simulink model "UberCase_cs"  (R2015b)
settings: Solver=ode5  SolverMode=SingleTasking  StartTime=0.0  StopTime=inf  FixedStep=1/100  RelTol=1e-3
PreLoadFcn:
  | mbxruntime.callbacks.PreLoadFcn(bdroot);
PostLoadFcn:
  | mbxruntime.callbacks.PostLoadFcn(bdroot);
InitFcn:
  | mbxruntime.callbacks.InitFcn(bdroot);
StartFcn:
  | mbxruntime.callbacks.StartFcn(bdroot);
StopFcn:
  | mbxruntime.callbacks.StopFcn(bdroot);
model workspace (MAT data in the model file):
  mbox_table : struct (value not decoded)
  model_closed = 0
  sim_status = 0
undefined symbols (not defined in the file or in its folder): DiscIntNeverNeededParam, InitImageOutputDir, mbxruntime, tabledata
libraries: PreScanSimulinkLibrary x32, simulink_extras x2, PreScanUsefulBlocks x1
(part 3 of 6)

== system UberCase_cs/STATE_Mazda_RX8_2_bus/ENABLED ==
  STATE_Mazda_RX8_2_bus : Inport  Tag=inport/StatePort  OutDataTypeStr=Bus: PRESCAN_STATEACTUATORDATA  PortDimensions=1  SampleTime=1/100  BusOutputAsStruct=on
  Actuator : S-Function  FunctionName=sfun_StateActuator  Parameters=UniqueID, TimeStep  SFunctionDeploymentMode=off  EnableBusSupport=off  mask(PreScan Sink Block: State){UniqueID=564, TimeStep=1/100}
      mask prompts: UniqueID "Auto-Assigned: Unique ID"; TimeStep "Auto-Assigned: Upload Period [s]"
      mask help:
      | The Actor State contains a vector signal of size (9x1), containing the following signals:
      |
      | -  Position    	(x,y,z)             	[m]
      | -  Velocity    	(vx,vy,vz)         	[m/s]
      | -  Angles       	(Roll, Pitch, Yaw)	[rad]
      |
      | The Actor state is defined in the global axis system.
      | The state is superponed on the Initial position defined in the GUI.
      |
      | For more information, please click Help.
      mask Help: eval('openHelp(222)')
      mask Display: image(imread('State.png'))
  wires:
  STATE_Mazda_RX8_2_bus/1 -> Actuator/1

== system UberCase_cs/STATE_Toyota_Previa_1_bus/DISABLED ==
  STATE_Toyota_Previa_1_bus : Inport  Tag=inport/StatePort  OutDataTypeStr=Bus: PRESCAN_STATEACTUATORDATA  PortDimensions=1  SampleTime=1/100  BusOutputAsStruct=on
  TRM1 : Terminator
  wires:
  STATE_Toyota_Previa_1_bus/1 -> TRM1/1

== system UberCase_cs/STATE_Toyota_Previa_1_bus/ENABLED ==
  STATE_Toyota_Previa_1_bus : Inport  Tag=inport/StatePort  OutDataTypeStr=Bus: PRESCAN_STATEACTUATORDATA  PortDimensions=1  SampleTime=1/100  BusOutputAsStruct=on
  Actuator : S-Function  FunctionName=sfun_StateActuator  Parameters=UniqueID, TimeStep  SFunctionDeploymentMode=off  EnableBusSupport=off  mask(PreScan Sink Block: State){UniqueID=665, TimeStep=1/100}
      mask prompts: UniqueID "Auto-Assigned: Unique ID"; TimeStep "Auto-Assigned: Upload Period [s]"
      mask help:
      | The Actor State contains a vector signal of size (9x1), containing the following signals:
      |
      | -  Position    	(x,y,z)             	[m]
      | -  Velocity    	(vx,vy,vz)         	[m/s]
      | -  Angles       	(Roll, Pitch, Yaw)	[rad]
      |
      | The Actor state is defined in the global axis system.
      | The state is superponed on the Initial position defined in the GUI.
      |
      | For more information, please click Help.
      mask Help: eval('openHelp(222)')
      mask Display: image(imread('State.png'))
  wires:
  STATE_Toyota_Previa_1_bus/1 -> Actuator/1

== system UberCase_cs/STATE_Uber_Car_bus/DISABLED ==
  STATE_Uber_Car_bus : Inport  Tag=inport/StatePort  OutDataTypeStr=Bus: PRESCAN_STATEACTUATORDATA  PortDimensions=1  SampleTime=1/100  BusOutputAsStruct=on
  TRM1 : Terminator
  wires:
  STATE_Uber_Car_bus/1 -> TRM1/1

== system UberCase_cs/STATE_Uber_Car_bus/ENABLED ==
  STATE_Uber_Car_bus : Inport  Tag=inport/StatePort  OutDataTypeStr=Bus: PRESCAN_STATEACTUATORDATA  PortDimensions=1  SampleTime=1/100  BusOutputAsStruct=on
  Actuator : S-Function  FunctionName=sfun_StateActuator  Parameters=UniqueID, TimeStep  SFunctionDeploymentMode=off  EnableBusSupport=off  mask(PreScan Sink Block: State){UniqueID=372, TimeStep=1/100}
      mask prompts: UniqueID "Auto-Assigned: Unique ID"; TimeStep "Auto-Assigned: Upload Period [s]"
      mask help:
      | The Actor State contains a vector signal of size (9x1), containing the following signals:
      |
      | -  Position    	(x,y,z)             	[m]
      | -  Velocity    	(vx,vy,vz)         	[m/s]
      | -  Angles       	(Roll, Pitch, Yaw)	[rad]
      |
      | The Actor state is defined in the global axis system.
      | The state is superponed on the Initial position defined in the GUI.
      |
      | For more information, please click Help.
      mask Help: eval('openHelp(222)')
      mask Display: image(imread('State.png'))
  wires:
  STATE_Uber_Car_bus/1 -> Actuator/1

== system UberCase_cs/Toyota_Previa_1/DISABLED ==
  SELF_Toyota_Previa_1 : Inport  Tag=inport/SelfPort  OutDataTypeStr=Bus: PRESCAN_SELFSENSORDATA  PortDimensions=1  SampleTime=1/100  BusOutputAsStruct=on
  GND1 : Subsystem
  TRM1 : Terminator
  STATE_Toyota_Previa_1_bus : Outport  Tag=outport/StatePort  OutDataTypeStr=Bus: PRESCAN_STATEACTUATORDATA  PortDimensions=1  SampleTime=1/100
  wires:
  SELF_Toyota_Previa_1/1 -> TRM1/1
  GND1/1(bus) -> STATE_Toyota_Previa_1_bus/1

== system UberCase_cs/Toyota_Previa_1/ENABLED ==
  SELF_Toyota_Previa_1 : Inport  Tag=inport/SelfPort  OutDataTypeStr=Bus: PRESCAN_SELFSENSORDATA  PortDimensions=1  SampleTime=1/100  BusOutputAsStruct=on
  Dynamics_Empty : Subsystem  Tag=Dynamics_Empty
      mask Help: eval('openHelp(202)')
      mask Display: port_label('output', 1, 'State');text(0,0,' Empty\n')
  SELF_Demux : Subsystem  Tag=demux/SelfPort  mask(PreScan Demux Block:){}
      mask help:
      | The SELF port shows (state) information of the actor itself. The outputs are position in the experiment's axis system and the GPS coordinates, and the object's absolute velocity and compass heading.
      |
      | For more information, please click Help.
      settings: DeleteFcn=PreScanBlockDeleteFcn;
      mask Help: eval('openHelp(462)')
      mask Display:
      | port_label('output',1,'x [m]')
      | port_label('output',2,'y [m]')
      | port_label('output',3,'z [m]','texmode','on')
      | port_label('output',4,'Rotx [deg]','texmode','on')
      | port_label('output',5,'Roty [deg]','texmode','on')
      | port_label('output',6,'Rotz [deg]','texmode','on')
      | port_label('output',7,'GPS lat [deg]','texmode','on')
      | port_label('output',8,'GPS long [deg]','texmode','on')
      | port_label('output',9,'GPS alt [m]','texmode','on')
      | port_label('output',10,'Velocity [m/s]')
      | port_label('output',11,'Heading [deg]')
      | port_label('output',12,'Yaw rate [deg/s]')
  STATE_Toyota_Previa_1 : Subsystem  Tag=mux/StatePort  Priority=0  LoadFcn=load PrescanStateActuatorData  mask(PreScan Sink Block: State){x0=82.046318054199219, y0=122.2374267578125, z0=0.71, Roll0=0, Pitch0=0, Yaw0=90, TimeStep=1/100}
      mask prompts: x0 "Ini x-position VEHICLE wrt GLOBAL axis system [m]"; y0 "Ini y-position VEHICLE wrt GLOBAL axis system [m]"; z0 "Ini z-position VEHICLE wrt GLOBAL axis system [m]"; Roll0 "Ini roll-angle BODY wrt VEHICLE axis system [deg]"; Pitch0 "Ini pitch-angle BODY wrt VEHICLE axis system [deg]"; Yaw0 "Ini yaw-angle VEHICLE wrt GLOBAL axis system [deg]"; TimeStep "Auto-Assigned: Upload Period [s]"
      mask help:
      | The Actor State contains a vector signal of size (9x1), containing the following signals:
      |
      | -  Position                  (x,y,z)                                     [m]
      | -  Velocity                  (vx,vy,vz)                               [m/s]
      | -  Angles                    (Roll, Pitch, Yaw)                   [rad]
      |
      | The Actor state is defined in the global axis system.
      | The state is superponed on the Initial position defined in the GUI.
      |
      | For more information, please click Help.
      settings: DeleteFcn=PreScanBlockDeleteFcn;
      mask Help: eval('openHelp(222)')
      mask Display: image(imread('State.png'))
  Terminator_{1..12} (12 alike) : Terminator
  STATE_Toyota_Previa_1_bus : Outport  Tag=outport/StatePort  OutDataTypeStr=Bus: PRESCAN_STATEACTUATORDATA  PortDimensions=1  SampleTime=1/100
  wires:
  STATE_Toyota_Previa_1/1(StateBus) -> STATE_Toyota_Previa_1_bus/1
  SELF_Toyota_Previa_1/1 -> SELF_Demux/1(SELF)
  Dynamics_Empty/1(State) -> STATE_Toyota_Previa_1/1(State)
  SELF_Demux/1(x [m]) -> Terminator_1/1
  SELF_Demux/2(y [m]) -> Terminator_2/1
  SELF_Demux/3(z [m]) -> Terminator_3/1
  SELF_Demux/4(rotx [deg]) -> Terminator_4/1
  SELF_Demux/5(roty [deg]) -> Terminator_5/1
  SELF_Demux/6(rotz [deg]) -> Terminator_6/1
  SELF_Demux/7(GPS lat [deg]) -> Terminator_7/1
  SELF_Demux/8(GPS long [deg]) -> Terminator_8/1
  SELF_Demux/9(GPS alt [m]) -> Terminator_9/1
  SELF_Demux/10(velocity [m/s]) -> Terminator_10/1
  SELF_Demux/11(heading [deg]) -> Terminator_11/1
  SELF_Demux/12(yaw rate [deg/s]) -> Terminator_12/1

== system UberCase_cs/TrafficLightSingleUS_1/DISABLED ==
  GND1 : Ground
  VISUCasingLights_TrafficLightSingleUS_1 : Outport  Tag=outport/VisuCasingLights  SampleTime=1/100
  wires:
  GND1/1 -> VISUCasingLights_TrafficLightSingleUS_1/1

== system UberCase_cs/TrafficLightSingleUS_1/ENABLED ==
  Ground_1 : Ground
  Ground_2 : Ground
  Ground_3 : Ground
  MATLAB Function : MATLAB Function  TreatAsAtomicUnit=on
  VISUCasingLights_Mux : Subsystem  Tag=mux/VisuCasingLights  mask(PreScan User Interface: VisuTrafficLight){}
      mask help:
      | The VisuTrafficLight block provides a way to animate traffic lights: switch on and off individual lights.
      |
      | For more information, please click Help.
      mask Help: eval('openHelp(731)')
  VISUCasingLights_TrafficLightSingleUS_1 : Outport  Tag=outport/VisuCasingLights  SampleTime=1/100
  wires:
  VISUCasingLights_Mux/1(VISUCasingLights_TrafficLightSingleUS_1) -> VISUCasingLights_TrafficLightSingleUS_1/1
  Ground_1/1 -> VISUCasingLights_Mux/1(Green [-])
  Ground_2/1 -> VISUCasingLights_Mux/2(Orange [-])
  Ground_3/1 -> VISUCasingLights_Mux/3(Red [-])

== system UberCase_cs/TrafficLightSingleUS_2/DISABLED ==
  GND1 : Ground
  VISUCasingLights_TrafficLightSingleUS_2 : Outport  Tag=outport/VisuCasingLights  SampleTime=1/100
  wires:
  GND1/1 -> VISUCasingLights_TrafficLightSingleUS_2/1

== system UberCase_cs/TrafficLightSingleUS_2/ENABLED ==
  Ground_1 : Ground
  Ground_2 : Ground
  Ground_3 : Ground
  VISUCasingLights_Mux : Subsystem  Tag=mux/VisuCasingLights  mask(PreScan User Interface: VisuTrafficLight){}
      mask help:
      | The VisuTrafficLight block provides a way to animate traffic lights: switch on and off individual lights.
      |
      | For more information, please click Help.
      mask Help: eval('openHelp(731)')
  VISUCasingLights_TrafficLightSingleUS_2 : Outport  Tag=outport/VisuCasingLights  SampleTime=1/100
  wires:
  VISUCasingLights_Mux/1(VISUCasingLights_TrafficLightSingleUS_2) -> VISUCasingLights_TrafficLightSingleUS_2/1
  Ground_1/1 -> VISUCasingLights_Mux/1(Green [-])
  Ground_2/1 -> VISUCasingLights_Mux/2(Orange [-])
  Ground_3/1 -> VISUCasingLights_Mux/3(Red [-])

== system UberCase_cs/Uber_Car/DISABLED ==
  SELF_Uber_Car : Inport  Tag=inport/SelfPort  OutDataTypeStr=Bus: PRESCAN_SELFSENSORDATA  PortDimensions=1  SampleTime=1/100  BusOutputAsStruct=on
  forward : Inport  Tag=inport/Camera/CameraSensor  Port=2  OutDataTypeStr=uint8  SampleTime=1/50  BusOutputAsStruct=on
  Lidar_Uber : Inport  Tag=inport/Lidar  Port=3  OutDataTypeStr=Bus: PRESCAN_SCANNERSENSOR_MESSAGE  PortDimensions=60  SampleTime=1/20  BusOutputAsStruct=on
  GND1 : Subsystem
  GND2 : Ground
  TRM1 : Terminator
  TRM2 : Terminator
  TRM3 : Terminator
  STATE_Uber_Car_bus : Outport  Tag=outport/StatePort  OutDataTypeStr=Bus: PRESCAN_STATEACTUATORDATA  PortDimensions=1  SampleTime=1/100
  VISUSteer_Uber_Car : Outport  Tag=outport/VisuSteer  Port=2  SampleTime=1/100
  wires:
  SELF_Uber_Car/1 -> TRM1/1
  forward/1 -> TRM2/1
  Lidar_Uber/1 -> TRM3/1
  GND1/1(bus) -> STATE_Uber_Car_bus/1
  GND2/1 -> VISUSteer_Uber_Car/1

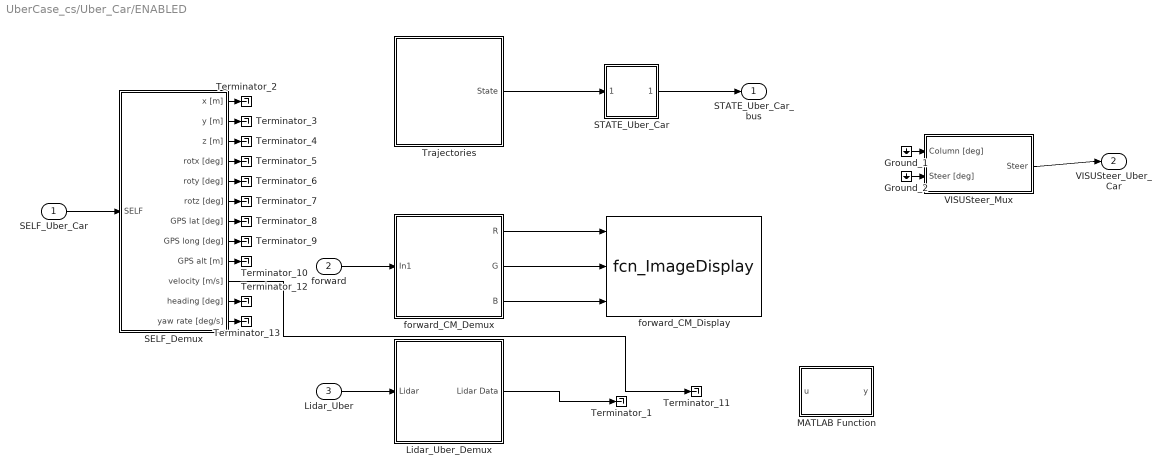
== system UberCase_cs/Uber_Car/ENABLED ==
  SELF_Uber_Car : Inport  Tag=inport/SelfPort  OutDataTypeStr=Bus: PRESCAN_SELFSENSORDATA  PortDimensions=1  SampleTime=1/100  BusOutputAsStruct=on
  forward : Inport  Tag=inport/Camera/CameraSensor  Port=2  OutDataTypeStr=uint8  SampleTime=1/50  BusOutputAsStruct=on
  Lidar_Uber : Inport  Tag=inport/Lidar  Port=3  OutDataTypeStr=Bus: PRESCAN_SCANNERSENSOR_MESSAGE  PortDimensions=60  SampleTime=1/20  BusOutputAsStruct=on
  Ground_1 : Ground
  Ground_2 : Ground
  Lidar_Uber_Demux : Subsystem  Tag=demux/Lidar  mask(PreScan Demux Block: Lidar){MAXMESSAGES=60}
      mask prompts: MAXMESSAGES "Number Of Objects"
      mask help:
      | The Lidar Sensor is a scanner device used to detect obstacles like cars, motor cycles, and pedestrians.
      |
      | For more information, please click Help.
      settings: DeleteFcn=PreScanBlockDeleteFcn;
      mask Help: eval('openHelp(1463)')
      mask Display:
      | port_label('input',1,'Lidar')
      | port_label('output',1,'Lidar Data')
  MATLAB Function : MATLAB Function  TreatAsAtomicUnit=on
  SELF_Demux : Subsystem  Tag=demux/SelfPort  mask(PreScan Demux Block:){}
      mask help:
      | The SELF port shows (state) information of the actor itself. The outputs are position in the experiment's axis system and the GPS coordinates, and the object's absolute velocity and compass heading.
      |
      | For more information, please click Help.
      settings: DeleteFcn=PreScanBlockDeleteFcn;
      mask Help: eval('openHelp(462)')
      mask Display:
      | port_label('output',1,'x [m]')
      | port_label('output',2,'y [m]')
      | port_label('output',3,'z [m]','texmode','on')
      | port_label('output',4,'Rotx [deg]','texmode','on')
      | port_label('output',5,'Roty [deg]','texmode','on')
      | port_label('output',6,'Rotz [deg]','texmode','on')
      | port_label('output',7,'GPS lat [deg]','texmode','on')
      | port_label('output',8,'GPS long [deg]','texmode','on')
      | port_label('output',9,'GPS alt [m]','texmode','on')
      | port_label('output',10,'Velocity [m/s]')
      | port_label('output',11,'Heading [deg]')
      | port_label('output',12,'Yaw rate [deg/s]')
  STATE_Uber_Car : Subsystem  Tag=mux/StatePort  Priority=0  LoadFcn=load PrescanStateActuatorData  mask(PreScan Sink Block: State){x0=85.2773666381836, y0=47.598899841308594, z0=0.55, Roll0=0, Pitch0=0, Yaw0=90.271814503097872, TimeStep=1/100}
      mask prompts: x0 "Ini x-position VEHICLE wrt GLOBAL axis system [m]"; y0 "Ini y-position VEHICLE wrt GLOBAL axis system [m]"; z0 "Ini z-position VEHICLE wrt GLOBAL axis system [m]"; Roll0 "Ini roll-angle BODY wrt VEHICLE axis system [deg]"; Pitch0 "Ini pitch-angle BODY wrt VEHICLE axis system [deg]"; Yaw0 "Ini yaw-angle VEHICLE wrt GLOBAL axis system [deg]"; TimeStep "Auto-Assigned: Upload Period [s]"
      mask help:
      | The Actor State contains a vector signal of size (9x1), containing the following signals:
      |
      | -  Position                  (x,y,z)                                     [m]
      | -  Velocity                  (vx,vy,vz)                               [m/s]
      | -  Angles                    (Roll, Pitch, Yaw)                   [rad]
      |
      | The Actor state is defined in the global axis system.
      | The state is superponed on the Initial position defined in the GUI.
      |
      | For more information, please click Help.
      settings: DeleteFcn=PreScanBlockDeleteFcn;
      mask Help: eval('openHelp(222)')
      mask Display: image(imread('State.png'))
  Terminator_{1..13} (13 alike) : Terminator
  Trajectories : Subsystem  Tag=Trajectories  mask(PreScan Source Block: Trajectories){}
      mask help:
      | The Trajectory block contains the trajectories defined in the PreScan Experiment Editor. The output of the trajectory block is the (vehicle) State.
      |
      | For more information, please click Help.
      settings: DeleteFcn=PreScanBlockDeleteFcn;
      mask Help: eval('openHelp(312)')
      mask Display: image(imread('Trajectory.png'));
  VISUSteer_Mux : Subsystem  Tag=mux/Steer_v2  mask(PreScan User Interface: VisuSteer){}
      mask help:
      | The VisuSteer block provides a way to adapt the orientation of the steering column and steering wheel of a vehicle.
      |
      | For more information, please click Help.
      settings: DeleteFcn=PreScanBlockDeleteFcn;
      mask Help: eval('openHelp(223)')
  forward_CM_Demux : Subsystem  Tag=demux/Camera/Color  mask{SensorName=forward, hres=500, vres=375}
      mask prompts: SensorName "Sensor Name"; hres "Horizontal Resolution"; vres "Vertical Resolution"
      mask Help: eval('openHelp(457)')
      mask Display:
      | fprintf('MONO CAMERA:\n Color\n %s \n %d x %d px',SensorName,hres,vres)
      | port_label('output',1,'R')
      | port_label('output',2,'G')
      | port_label('output',3,'B')
  forward_CM_Display : M-S-Function  Tag=CameraSensor_Color_Display  InitFcn=InitImageOutputDir(gcb);  FunctionName=fcn_ImageDisplay  Parameters=SensorName EnableDisplay EnablePosition DisplayPosition FigureHandle SaveResults BitmapFormat TempOutputDir CameraType DataType  mask(PreScan Color Display Block){SensorName=forward, EnableDisplay=on, EnablePosition=off, DisplayPosition=[10 10 500 375], FigureHandle=37201, SaveResults=off, Format=PNG, TempOutputDir=0, CameraType=Mono, DataType=uint8}
      mask prompts: SensorName "User Specified: Title of Display"; EnableDisplay "Active"; EnablePosition "Set Display window position"; DisplayPosition "Display window position [xpos ypos width height]"; FigureHandle "Unique Handle"; SaveResults "Save results"; TempOutputDir "OutputDir"; CameraType "Camera Type"; DataType "Image Data Type"
      mask help: This block displays the RGB output of a PreScan camera sensor.
      mask init: same as UberCase_cs/Conventional_Car/ENABLED/Camera_conventional_CM_Display
      settings: CopyFcn=CopyFcnDisplay  DeleteFcn=PreScanBlockDeleteFcn;  ModelCloseFcn=fcn_ImageDisplay_ModelCloseFcn
      mask Help: eval('openHelp(457)')
      mask Callback EnablePosition:
      | MV=get_param(gcb,'MaskVisibilities');
      | if strcmp(get_param(gcb,'EnablePosition'),'on')
      |     MV{4}='on';
      | else
      |     MV{4}='off';
      | end
      | set_param(gcb,'MaskVisibilities',MV);
      | clear MV;
      mask TypeOptions Format: PNG | BMP | JPG
      mask TypeOptions CameraType: Mono | Stereo
      mask TypeOptions DataType: uint8 | single
      mask Display:
      | color(EnableColor);
      | fprintf('%s\n DISPLAY:\n Color \n %s',EnableString,SensorName)
      | port_label('input',1,'R')
      | port_label('input',2,'G')
      | port_label('input',3,'B')
      | port_label('input',PortNumber+1,'R')
      | port_label('input',PortNumber+2,'G')
      | port_label('input',PortNumber+3,'B')
  STATE_Uber_Car_bus : Outport  Tag=outport/StatePort  OutDataTypeStr=Bus: PRESCAN_STATEACTUATORDATA  PortDimensions=1  SampleTime=1/100
  VISUSteer_Uber_Car : Outport  Tag=outport/VisuSteer  Port=2  SampleTime=1/100
  wires:
  STATE_Uber_Car/1(StateBus) -> STATE_Uber_Car_bus/1
  SELF_Uber_Car/1 -> SELF_Demux/1(SELF)
  forward/1 -> forward_CM_Demux/1(In1)
  forward_CM_Demux/1(R) -> forward_CM_Display/1
  forward_CM_Demux/2(G) -> forward_CM_Display/2
  forward_CM_Demux/3(B) -> forward_CM_Display/3
  Lidar_Uber/1 -> Lidar_Uber_Demux/1(Lidar)
  VISUSteer_Mux/1(Steer) -> VISUSteer_Uber_Car/1
  Trajectories/1(State) -> STATE_Uber_Car/1(State)
  Lidar_Uber_Demux/1(Lidar Data) -> Terminator_1/1
  SELF_Demux/1(x [m]) -> Terminator_2/1
  SELF_Demux/2(y [m]) -> Terminator_3/1
  SELF_Demux/3(z [m]) -> Terminator_4/1
  SELF_Demux/4(rotx [deg]) -> Terminator_5/1
  SELF_Demux/5(roty [deg]) -> Terminator_6/1
  SELF_Demux/6(rotz [deg]) -> Terminator_7/1
  SELF_Demux/7(GPS lat [deg]) -> Terminator_8/1
  SELF_Demux/8(GPS long [deg]) -> Terminator_9/1
  SELF_Demux/9(GPS alt [m]) -> Terminator_10/1
  SELF_Demux/10(velocity [m/s]) -> Terminator_11/1
  SELF_Demux/11(heading [deg]) -> Terminator_12/1
  SELF_Demux/12(yaw rate [deg/s]) -> Terminator_13/1
  Ground_1/1 -> VISUSteer_Mux/1(Column [deg])
  Ground_2/1 -> VISUSteer_Mux/2(Steer [deg])

== system UberCase_cs/VISUCasingLights_TrafficLightSingleUS_1/DISABLED ==
  VISUCasingLights_TrafficLightSingleUS_1 : Inport  Tag=inport/VisuCasingLights  SampleTime=1/100  BusOutputAsStruct=on
  TRM1 : Terminator
  wires:
  VISUCasingLights_TrafficLightSingleUS_1/1 -> TRM1/1

== system UberCase_cs/VISUCasingLights_TrafficLightSingleUS_1/ENABLED ==
  VISUCasingLights_TrafficLightSingleUS_1 : Inport  Tag=inport/VisuCasingLights  SampleTime=1/100  BusOutputAsStruct=on
  Actuator : Subsystem  mask(PreScan Sink Block: VisuTrafficLight){UniqueID=704, ColorsObjectQuery=, Colors=[]}
      mask prompts: UniqueID "Parent Unique Identifier"; ColorsObjectQuery "Query for Color Object"; Colors "Matrix of colors"
      mask help:
      | The VisuTrafficLight block provides a way to animate traffic lights: switch on and off individual lights.
      |
      | For more information, please click Help.
      mask Help: eval('openHelp(731)')
      mask Display: image(imread('TrafficLightCasing.png'))
  wires:
  VISUCasingLights_TrafficLightSingleUS_1/1 -> Actuator/1(VISUCasingLights_TrafficLightSingleUS_1)

== system UberCase_cs/VISUCasingLights_TrafficLightSingleUS_2/DISABLED ==
  VISUCasingLights_TrafficLightSingleUS_2 : Inport  Tag=inport/VisuCasingLights  SampleTime=1/100  BusOutputAsStruct=on
  TRM1 : Terminator
  wires:
  VISUCasingLights_TrafficLightSingleUS_2/1 -> TRM1/1

== system UberCase_cs/VISUCasingLights_TrafficLightSingleUS_2/ENABLED ==
  VISUCasingLights_TrafficLightSingleUS_2 : Inport  Tag=inport/VisuCasingLights  SampleTime=1/100  BusOutputAsStruct=on
  Actuator : Subsystem  mask(PreScan Sink Block: VisuTrafficLight){UniqueID=705, ColorsObjectQuery=, Colors=[]}
      mask prompts: UniqueID "Parent Unique Identifier"; ColorsObjectQuery "Query for Color Object"; Colors "Matrix of colors"
      mask help:
      | The VisuTrafficLight block provides a way to animate traffic lights: switch on and off individual lights.
      |
      | For more information, please click Help.
      mask Help: eval('openHelp(731)')
      mask Display: image(imread('TrafficLightCasing.png'))
  wires:
  VISUCasingLights_TrafficLightSingleUS_2/1 -> Actuator/1(VISUCasingLights_TrafficLightSingleUS_2)

== system UberCase_cs/VISUSteer_Conventional_Car/DISABLED ==
  VISUSteer_Conventional_Car : Inport  Tag=inport/VisuSteer  SampleTime=1/100  BusOutputAsStruct=on
  TRM1 : Terminator
  wires:
  VISUSteer_Conventional_Car/1 -> TRM1/1

== system UberCase_cs/VISUSteer_Conventional_Car/ENABLED ==
  VISUSteer_Conventional_Car : Inport  Tag=inport/VisuSteer  SampleTime=1/100  BusOutputAsStruct=on
  Actuator : Subsystem  Tag=VisuSteer  VariantControl=on  mask(PreScan Sink Block: VisuSteer){UniqueID=371, ObjectName=Conventional_Car, TimeStep=1/100}
      mask prompts: UniqueID "Auto-Assigned: Parent Unique ID"; ObjectName "Auto-Assigned: Parent Object Name"; TimeStep "Auto-Assigned: Upload Period [s]"
      mask help:
      | The VisuSteer block provides a way to adapt the orientation of the steering column and steering wheel of a vehicle.
      |
      | For more information, please click Help.
      settings: DeleteFcn=PreScanBlockDeleteFcn;
      mask Help: eval('openHelp(223)')
      mask Display: image(imread('steeringwheel.png'))
  wires:
  VISUSteer_Conventional_Car/1 -> Actuator/1(SteerInput)

== system UberCase_cs/VISUSteer_Uber_Car/DISABLED ==
  VISUSteer_Uber_Car : Inport  Tag=inport/VisuSteer  SampleTime=1/100  BusOutputAsStruct=on
  TRM1 : Terminator
  wires:
  VISUSteer_Uber_Car/1 -> TRM1/1

== system UberCase_cs/VISUSteer_Uber_Car/ENABLED ==
  VISUSteer_Uber_Car : Inport  Tag=inport/VisuSteer  SampleTime=1/100  BusOutputAsStruct=on
  Actuator : Subsystem  Tag=VisuSteer  VariantControl=on  mask(PreScan Sink Block: VisuSteer){UniqueID=372, ObjectName=Uber_Car, TimeStep=1/100}
      mask prompts: UniqueID "Auto-Assigned: Parent Unique ID"; ObjectName "Auto-Assigned: Parent Object Name"; TimeStep "Auto-Assigned: Upload Period [s]"
      mask help:
      | The VisuSteer block provides a way to adapt the orientation of the steering column and steering wheel of a vehicle.
      |
      | For more information, please click Help.
      settings: DeleteFcn=PreScanBlockDeleteFcn;
      mask Help: eval('openHelp(223)')
      mask Display: image(imread('steeringwheel.png'))
  wires:
  VISUSteer_Uber_Car/1 -> Actuator/1(SteerInput)

== system UberCase_cs/forward/DISABLED ==
  GND1 : Ground
  forward : Outport  Tag=outport/Camera/CameraSensor  OutDataTypeStr=uint8  SampleTime=1/50
  wires:
  GND1/1 -> forward/1

== system UberCase_cs/forward/ENABLED ==
  Sensor : S-Function  FunctionName=sfun_Camera  Parameters=sensorID, dataWidth, dataHeight, channelsPerImage, numberOfImages, timestep  SFunctionDeploymentMode=off  EnableBusSupport=off  mask(PreScan Source Block: Camera Sensor){sensorID=373, dataWidth=375, dataHeight=1500, channelsPerImage=3, numberOfImages=1, timestep=1/50}
      mask prompts: sensorID "Sensor ID"; dataWidth "Data width"; dataHeight "Data Height"; channelsPerImage "Channels per image"; numberOfImages "Number of images"; timestep "MATLAB timestep:"
      mask help: The Camera Sensor provides a color or monochrome image.
      mask Help: eval('openHelp(457)')
      mask Display: image(imread('CameraSensor.png'))
  forward : Outport  Tag=outport/Camera/CameraSensor  OutDataTypeStr=uint8  SampleTime=1/50
  wires:
  Sensor/1 -> forward/1

== system UberCase_cs/Audi_A8_1/DISABLED/GND1 ==
  GND_AccelerationX : Constant  Value=0
  GND_AccelerationY : Constant  Value=0
  GND_AccelerationZ : Constant  Value=0
  GND_AngularVelocityPitch : Constant  Value=0
  GND_AngularVelocityRoll : Constant  Value=0
  GND_AngularVelocityYaw : Constant  Value=0
  GND_OrientationPitch : Constant  Value=0
  GND_OrientationRoll : Constant  Value=0
  GND_OrientationYaw : Constant  Value=0
  GND_PositionX : Constant  Value=0
  GND_PositionY : Constant  Value=0
  GND_PositionZ : Constant  Value=0
  GND_VelocityX : Constant  Value=0
  GND_VelocityY : Constant  Value=0
  GND_VelocityZ : Constant  Value=0
  buscreator : BusCreator  Inputs=15  OutDataTypeStr=Bus: PRESCAN_STATEACTUATORDATA  NonVirtualBus=on
  bus : Outport  OutDataTypeStr=Bus: PRESCAN_STATEACTUATORDATA
  wires:
  GND_PositionX/1 -> buscreator/1  "PositionX"
  GND_PositionY/1 -> buscreator/2  "PositionY"
  GND_PositionZ/1 -> buscreator/3  "PositionZ"
  GND_VelocityX/1 -> buscreator/4  "VelocityX"
  GND_VelocityY/1 -> buscreator/5  "VelocityY"
  GND_VelocityZ/1 -> buscreator/6  "VelocityZ"
  GND_AccelerationX/1 -> buscreator/7  "AccelerationX"
  GND_AccelerationY/1 -> buscreator/8  "AccelerationY"
  GND_AccelerationZ/1 -> buscreator/9  "AccelerationZ"
  GND_OrientationRoll/1 -> buscreator/10  "OrientationRoll"
  GND_OrientationPitch/1 -> buscreator/11  "OrientationPitch"
  GND_OrientationYaw/1 -> buscreator/12  "OrientationYaw"
  GND_AngularVelocityRoll/1 -> buscreator/13  "AngularVelocityRoll"
  GND_AngularVelocityPitch/1 -> buscreator/14  "AngularVelocityPitch"
  GND_AngularVelocityYaw/1 -> buscreator/15  "AngularVelocityYaw"
  buscreator/1 -> bus/1

== system UberCase_cs/Audi_A8_1/ENABLED/Dynamics_Empty ==
  note: For state mode 'Dynamic' positions
      | are not taken into account, as they
      | are computed by integrating velocity.
      | Click annotation for Help.
  Ground_{1..9} (9 alike) : Ground
  MuxState : Subsystem  Tag=mux/State  mask(Empty Dynamics State Block){positioningmode=on, TimeStep=1/100}
      mask prompts: positioningmode "Positioning Mode"; TimeStep "Auto Assigned: Time Step [s]"
      mask help:
      | Build the state of an actor based on user input.
      | The user can either use positioning mode or dynamics mode.
      | - When using positioning mode the position and orientation of the actor are set directly based on the input. Expected input is relative to the initial position and orientation of the actor. It's also possible to specify the velocity of the actor, though this input isn't used, only passed on.
      | - When using dynamics mode the position input is ignored. Expected input is velocity and orientation. The velocity is relative the current orientation of the actor, while orientation is relative to its initial orientation. The position of the actor is calculated based on the velocity and orientation given.
      settings: DeleteFcn=PreScanBlockDeleteFcn;
  State : Outport  Tag=outport/StateOutport  SampleTime=1/100
  wires:
  MuxState/1(state) -> State/1
  Ground_1/1 -> MuxState/1(x [m])
  Ground_2/1 -> MuxState/2(y [m])
  Ground_3/1 -> MuxState/3(z [m])
  Ground_4/1 -> MuxState/4(dx [m/s])
  Ground_5/1 -> MuxState/5(dy [m/s])
  Ground_6/1 -> MuxState/6(dz [m/s])
  Ground_7/1 -> MuxState/7(R [rad])
  Ground_8/1 -> MuxState/8(P [rad])
  Ground_9/1 -> MuxState/9(Y [rad])

== system UberCase_cs/Audi_A8_1/ENABLED/SELF_Demux ==
  SELF : Inport  OutDataTypeStr=Bus: PRESCAN_SELFSENSORDATA
  Bus Selector : BusSelector  OutputSignals=PositionX,PositionY,PositionZ,OrientationRoll,OrientationPitch,OrientationYaw,Velocity,Yaw_rate,Lat,Long,Alt
  Demux2 : Demux  Outputs=3
  Gain : Gain  Gain=180/pi
  Gain1 : Gain  Gain=180/pi
  Vector Concatenate1 : Concatenate  NumInputs=3
  compas converter : Subsystem
  x [m] : Outport
  y [m] : Outport  Port=2
  z [m] : Outport  Port=3
  rotx [deg] : Outport  Port=4
  roty [deg] : Outport  Port=5
  rotz [deg] : Outport  Port=6
  GPS lat [deg] : Outport  Port=7
  GPS long [deg] : Outport  Port=8
  GPS alt [m] : Outport  Port=9
  velocity [m/s] : Outport  Port=10
  heading [deg] : Outport  Port=11
  yaw rate [deg/s] : Outport  Port=12
  wires:
  Bus Selector/11 -> GPS alt [m]/1  "<Alt>"
  Bus Selector/10 -> GPS long [deg]/1  "<Long>"
  Bus Selector/9 -> GPS lat [deg]/1  "<Lat>"
  Bus Selector/8 -> Gain1/1  "<Yaw_rate>"
  Bus Selector/7 -> velocity [m/s]/1  "<Velocity>"
  Bus Selector/6 -> compas converter/1(rotz [rad]), Vector Concatenate1/3  "<OrientationYaw>"
  Bus Selector/5 -> Vector Concatenate1/2  "<OrientationPitch>"
  Bus Selector/4 -> Vector Concatenate1/1  "<OrientationRoll>"
  Vector Concatenate1/1 -> Gain/1
  Bus Selector/3 -> z [m]/1  "<PositionZ>"
  Bus Selector/2 -> y [m]/1  "<PositionY>"
  Bus Selector/1 -> x [m]/1  "<PositionX>"
  SELF/1 -> Bus Selector/1
  Gain/1 -> Demux2/1
  Demux2/1 -> rotx [deg]/1
  Demux2/2 -> roty [deg]/1
  Demux2/3 -> rotz [deg]/1
  compas converter/1(heading [deg]) -> heading [deg]/1
  Gain1/1 -> yaw rate [deg/s]/1

== system UberCase_cs/Audi_A8_1/ENABLED/STATE_Audi_A8_1 ==
  State : Inport  SampleTime=TimeStep
  Bus Creator : BusCreator  Inputs=15  OutDataTypeStr=Bus: PRESCAN_STATEACTUATORDATA  NonVirtualBus=on
  Demux : Demux  Outputs=15
  iniBODYAngles wrtVEH [rad] : Constant  Value=[Roll0 Pitch0 0]  SampleTime=TimeStep
  iniVEHAngles wrtGLOB [rad] : Constant  Value=[0 0 Yaw0]  SampleTime=TimeStep
  iniVEHposition wrtGLOB [m] : Constant  Value=[x0 y0 z0]  SampleTime=TimeStep
  state2FullState : PreScanSimulinkLibrary/state2FullState  SystemSampleTime=-1
  StateBus : Outport  OutDataTypeStr=Bus: PRESCAN_STATEACTUATORDATA
  wires:
  Bus Creator/1 -> StateBus/1
  State/1 -> state2FullState/1
  state2FullState/1 -> Demux/1
  iniVEHposition wrtGLOB [m]/1 -> state2FullState/2
  iniBODYAngles wrtVEH [rad]/1 -> state2FullState/3
  iniVEHAngles wrtGLOB [rad]/1 -> state2FullState/4
  Demux/1 -> Bus Creator/1  "PositionX"
  Demux/2 -> Bus Creator/2  "PositionY"
  Demux/3 -> Bus Creator/3  "PositionZ"
  Demux/4 -> Bus Creator/4  "VelocityX"
  Demux/5 -> Bus Creator/5  "VelocityY"
  Demux/6 -> Bus Creator/6  "VelocityZ"
  Demux/7 -> Bus Creator/7  "AccelerationX"
  Demux/8 -> Bus Creator/8  "AccelerationY"
  Demux/9 -> Bus Creator/9  "AccelerationZ"
  Demux/10 -> Bus Creator/10  "OrientationRoll"
  Demux/11 -> Bus Creator/11  "OrientationPitch"
  Demux/12 -> Bus Creator/12  "OrientationYaw"
  Demux/13 -> Bus Creator/13  "AngularVelocityRoll"
  Demux/14 -> Bus Creator/14  "AngularVelocityPitch"
  Demux/15 -> Bus Creator/15  "AngularVelocityYaw"

== system UberCase_cs/Audi_A8_2/DISABLED/GND1 ==
  GND_AccelerationX : Constant  Value=0
  GND_AccelerationY : Constant  Value=0
  GND_AccelerationZ : Constant  Value=0
  GND_AngularVelocityPitch : Constant  Value=0
  GND_AngularVelocityRoll : Constant  Value=0
  GND_AngularVelocityYaw : Constant  Value=0
  GND_OrientationPitch : Constant  Value=0
  GND_OrientationRoll : Constant  Value=0
  GND_OrientationYaw : Constant  Value=0
  GND_PositionX : Constant  Value=0
  GND_PositionY : Constant  Value=0
  GND_PositionZ : Constant  Value=0
  GND_VelocityX : Constant  Value=0
  GND_VelocityY : Constant  Value=0
  GND_VelocityZ : Constant  Value=0
  buscreator : BusCreator  Inputs=15  OutDataTypeStr=Bus: PRESCAN_STATEACTUATORDATA  NonVirtualBus=on
  bus : Outport  OutDataTypeStr=Bus: PRESCAN_STATEACTUATORDATA
  wires:
  GND_PositionX/1 -> buscreator/1  "PositionX"
  GND_PositionY/1 -> buscreator/2  "PositionY"
  GND_PositionZ/1 -> buscreator/3  "PositionZ"
  GND_VelocityX/1 -> buscreator/4  "VelocityX"
  GND_VelocityY/1 -> buscreator/5  "VelocityY"
  GND_VelocityZ/1 -> buscreator/6  "VelocityZ"
  GND_AccelerationX/1 -> buscreator/7  "AccelerationX"
  GND_AccelerationY/1 -> buscreator/8  "AccelerationY"
  GND_AccelerationZ/1 -> buscreator/9  "AccelerationZ"
  GND_OrientationRoll/1 -> buscreator/10  "OrientationRoll"
  GND_OrientationPitch/1 -> buscreator/11  "OrientationPitch"
  GND_OrientationYaw/1 -> buscreator/12  "OrientationYaw"
  GND_AngularVelocityRoll/1 -> buscreator/13  "AngularVelocityRoll"
  GND_AngularVelocityPitch/1 -> buscreator/14  "AngularVelocityPitch"
  GND_AngularVelocityYaw/1 -> buscreator/15  "AngularVelocityYaw"
  buscreator/1 -> bus/1

== system UberCase_cs/Audi_A8_2/ENABLED/Dynamics_Empty ==
  note: For state mode 'Dynamic' positions
      | are not taken into account, as they
      | are computed by integrating velocity.
      | Click annotation for Help.
  Ground_{1..9} (9 alike) : Ground
  MuxState : Subsystem  Tag=mux/State  mask(Empty Dynamics State Block){positioningmode=on, TimeStep=1/100}
      mask prompts: positioningmode "Positioning Mode"; TimeStep "Auto Assigned: Time Step [s]"
      mask help:
      | Build the state of an actor based on user input.
      | The user can either use positioning mode or dynamics mode.
      | - When using positioning mode the position and orientation of the actor are set directly based on the input. Expected input is relative to the initial position and orientation of the actor. It's also possible to specify the velocity of the actor, though this input isn't used, only passed on.
      | - When using dynamics mode the position input is ignored. Expected input is velocity and orientation. The velocity is relative the current orientation of the actor, while orientation is relative to its initial orientation. The position of the actor is calculated based on the velocity and orientation given.
      settings: DeleteFcn=PreScanBlockDeleteFcn;
  State : Outport  Tag=outport/StateOutport  SampleTime=1/100
  wires:
  MuxState/1(state) -> State/1
  Ground_1/1 -> MuxState/1(x [m])
  Ground_2/1 -> MuxState/2(y [m])
  Ground_3/1 -> MuxState/3(z [m])
  Ground_4/1 -> MuxState/4(dx [m/s])
  Ground_5/1 -> MuxState/5(dy [m/s])
  Ground_6/1 -> MuxState/6(dz [m/s])
  Ground_7/1 -> MuxState/7(R [rad])
  Ground_8/1 -> MuxState/8(P [rad])
  Ground_9/1 -> MuxState/9(Y [rad])

== system UberCase_cs/Audi_A8_2/ENABLED/SELF_Demux ==
  SELF : Inport  OutDataTypeStr=Bus: PRESCAN_SELFSENSORDATA
  Bus Selector : BusSelector  OutputSignals=PositionX,PositionY,PositionZ,OrientationRoll,OrientationPitch,OrientationYaw,Velocity,Yaw_rate,Lat,Long,Alt
  Demux2 : Demux  Outputs=3
  Gain : Gain  Gain=180/pi
  Gain1 : Gain  Gain=180/pi
  Vector Concatenate1 : Concatenate  NumInputs=3
  compas converter : Subsystem
  x [m] : Outport
  y [m] : Outport  Port=2
  z [m] : Outport  Port=3
  rotx [deg] : Outport  Port=4
  roty [deg] : Outport  Port=5
  rotz [deg] : Outport  Port=6
  GPS lat [deg] : Outport  Port=7
  GPS long [deg] : Outport  Port=8
  GPS alt [m] : Outport  Port=9
  velocity [m/s] : Outport  Port=10
  heading [deg] : Outport  Port=11
  yaw rate [deg/s] : Outport  Port=12
  wires:
  Bus Selector/11 -> GPS alt [m]/1  "<Alt>"
  Bus Selector/10 -> GPS long [deg]/1  "<Long>"
  Bus Selector/9 -> GPS lat [deg]/1  "<Lat>"
  Bus Selector/8 -> Gain1/1  "<Yaw_rate>"
  Bus Selector/7 -> velocity [m/s]/1  "<Velocity>"
  Bus Selector/6 -> compas converter/1(rotz [rad]), Vector Concatenate1/3  "<OrientationYaw>"
  Bus Selector/5 -> Vector Concatenate1/2  "<OrientationPitch>"
  Bus Selector/4 -> Vector Concatenate1/1  "<OrientationRoll>"
  Vector Concatenate1/1 -> Gain/1
  Bus Selector/3 -> z [m]/1  "<PositionZ>"
  Bus Selector/2 -> y [m]/1  "<PositionY>"
  Bus Selector/1 -> x [m]/1  "<PositionX>"
  SELF/1 -> Bus Selector/1
  Gain/1 -> Demux2/1
  Demux2/1 -> rotx [deg]/1
  Demux2/2 -> roty [deg]/1
  Demux2/3 -> rotz [deg]/1
  compas converter/1(heading [deg]) -> heading [deg]/1
  Gain1/1 -> yaw rate [deg/s]/1

== system UberCase_cs/Audi_A8_2/ENABLED/STATE_Audi_A8_2 ==
  State : Inport  SampleTime=TimeStep
  Bus Creator : BusCreator  Inputs=15  OutDataTypeStr=Bus: PRESCAN_STATEACTUATORDATA  NonVirtualBus=on
  Demux : Demux  Outputs=15
  iniBODYAngles wrtVEH [rad] : Constant  Value=[Roll0 Pitch0 0]  SampleTime=TimeStep
  iniVEHAngles wrtGLOB [rad] : Constant  Value=[0 0 Yaw0]  SampleTime=TimeStep
  iniVEHposition wrtGLOB [m] : Constant  Value=[x0 y0 z0]  SampleTime=TimeStep
  state2FullState : PreScanSimulinkLibrary/state2FullState  SystemSampleTime=-1
  StateBus : Outport  OutDataTypeStr=Bus: PRESCAN_STATEACTUATORDATA
  wires:
  Bus Creator/1 -> StateBus/1
  State/1 -> state2FullState/1
  state2FullState/1 -> Demux/1
  iniVEHposition wrtGLOB [m]/1 -> state2FullState/2
  iniBODYAngles wrtVEH [rad]/1 -> state2FullState/3
  iniVEHAngles wrtGLOB [rad]/1 -> state2FullState/4
  Demux/1 -> Bus Creator/1  "PositionX"
  Demux/2 -> Bus Creator/2  "PositionY"
  Demux/3 -> Bus Creator/3  "PositionZ"
  Demux/4 -> Bus Creator/4  "VelocityX"
  Demux/5 -> Bus Creator/5  "VelocityY"
  Demux/6 -> Bus Creator/6  "VelocityZ"
  Demux/7 -> Bus Creator/7  "AccelerationX"
  Demux/8 -> Bus Creator/8  "AccelerationY"
  Demux/9 -> Bus Creator/9  "AccelerationZ"
  Demux/10 -> Bus Creator/10  "OrientationRoll"
  Demux/11 -> Bus Creator/11  "OrientationPitch"
  Demux/12 -> Bus Creator/12  "OrientationYaw"
  Demux/13 -> Bus Creator/13  "AngularVelocityRoll"
  Demux/14 -> Bus Creator/14  "AngularVelocityPitch"
  Demux/15 -> Bus Creator/15  "AngularVelocityYaw"

== system UberCase_cs/BMW_X5_1/DISABLED/GND1 ==
  GND_AccelerationX : Constant  Value=0
  GND_AccelerationY : Constant  Value=0
  GND_AccelerationZ : Constant  Value=0
  GND_AngularVelocityPitch : Constant  Value=0
  GND_AngularVelocityRoll : Constant  Value=0
  GND_AngularVelocityYaw : Constant  Value=0
  GND_OrientationPitch : Constant  Value=0
  GND_OrientationRoll : Constant  Value=0
  GND_OrientationYaw : Constant  Value=0
  GND_PositionX : Constant  Value=0
  GND_PositionY : Constant  Value=0
  GND_PositionZ : Constant  Value=0
  GND_VelocityX : Constant  Value=0
  GND_VelocityY : Constant  Value=0
  GND_VelocityZ : Constant  Value=0
  buscreator : BusCreator  Inputs=15  OutDataTypeStr=Bus: PRESCAN_STATEACTUATORDATA  NonVirtualBus=on
  bus : Outport  OutDataTypeStr=Bus: PRESCAN_STATEACTUATORDATA
  wires:
  GND_PositionX/1 -> buscreator/1  "PositionX"
  GND_PositionY/1 -> buscreator/2  "PositionY"
  GND_PositionZ/1 -> buscreator/3  "PositionZ"
  GND_VelocityX/1 -> buscreator/4  "VelocityX"
  GND_VelocityY/1 -> buscreator/5  "VelocityY"
  GND_VelocityZ/1 -> buscreator/6  "VelocityZ"
  GND_AccelerationX/1 -> buscreator/7  "AccelerationX"
  GND_AccelerationY/1 -> buscreator/8  "AccelerationY"
  GND_AccelerationZ/1 -> buscreator/9  "AccelerationZ"
  GND_OrientationRoll/1 -> buscreator/10  "OrientationRoll"
  GND_OrientationPitch/1 -> buscreator/11  "OrientationPitch"
  GND_OrientationYaw/1 -> buscreator/12  "OrientationYaw"
  GND_AngularVelocityRoll/1 -> buscreator/13  "AngularVelocityRoll"
  GND_AngularVelocityPitch/1 -> buscreator/14  "AngularVelocityPitch"
  GND_AngularVelocityYaw/1 -> buscreator/15  "AngularVelocityYaw"
  buscreator/1 -> bus/1

== system UberCase_cs/BMW_X5_1/ENABLED/Dynamics_Empty ==
  note: For state mode 'Dynamic' positions
      | are not taken into account, as they
      | are computed by integrating velocity.
      | Click annotation for Help.
  Ground_{1..9} (9 alike) : Ground
  MuxState : Subsystem  Tag=mux/State  mask(Empty Dynamics State Block){positioningmode=on, TimeStep=1/100}
      mask prompts: positioningmode "Positioning Mode"; TimeStep "Auto Assigned: Time Step [s]"
      mask help:
      | Build the state of an actor based on user input.
      | The user can either use positioning mode or dynamics mode.
      | - When using positioning mode the position and orientation of the actor are set directly based on the input. Expected input is relative to the initial position and orientation of the actor. It's also possible to specify the velocity of the actor, though this input isn't used, only passed on.
      | - When using dynamics mode the position input is ignored. Expected input is velocity and orientation. The velocity is relative the current orientation of the actor, while orientation is relative to its initial orientation. The position of the actor is calculated based on the velocity and orientation given.
      settings: DeleteFcn=PreScanBlockDeleteFcn;
  State : Outport  Tag=outport/StateOutport  SampleTime=1/100
  wires:
  MuxState/1(state) -> State/1
  Ground_1/1 -> MuxState/1(x [m])
  Ground_2/1 -> MuxState/2(y [m])
  Ground_3/1 -> MuxState/3(z [m])
  Ground_4/1 -> MuxState/4(dx [m/s])
  Ground_5/1 -> MuxState/5(dy [m/s])
  Ground_6/1 -> MuxState/6(dz [m/s])
  Ground_7/1 -> MuxState/7(R [rad])
  Ground_8/1 -> MuxState/8(P [rad])
  Ground_9/1 -> MuxState/9(Y [rad])

== system UberCase_cs/BMW_X5_1/ENABLED/SELF_Demux ==
  SELF : Inport  OutDataTypeStr=Bus: PRESCAN_SELFSENSORDATA
  Bus Selector : BusSelector  OutputSignals=PositionX,PositionY,PositionZ,OrientationRoll,OrientationPitch,OrientationYaw,Velocity,Yaw_rate,Lat,Long,Alt
  Demux2 : Demux  Outputs=3
  Gain : Gain  Gain=180/pi
  Gain1 : Gain  Gain=180/pi
  Vector Concatenate1 : Concatenate  NumInputs=3
  compas converter : Subsystem
  x [m] : Outport
  y [m] : Outport  Port=2
  z [m] : Outport  Port=3
  rotx [deg] : Outport  Port=4
  roty [deg] : Outport  Port=5
  rotz [deg] : Outport  Port=6
  GPS lat [deg] : Outport  Port=7
  GPS long [deg] : Outport  Port=8
  GPS alt [m] : Outport  Port=9
  velocity [m/s] : Outport  Port=10
  heading [deg] : Outport  Port=11
  yaw rate [deg/s] : Outport  Port=12
  wires:
  Bus Selector/11 -> GPS alt [m]/1  "<Alt>"
  Bus Selector/10 -> GPS long [deg]/1  "<Long>"
  Bus Selector/9 -> GPS lat [deg]/1  "<Lat>"
  Bus Selector/8 -> Gain1/1  "<Yaw_rate>"
  Bus Selector/7 -> velocity [m/s]/1  "<Velocity>"
  Bus Selector/6 -> compas converter/1(rotz [rad]), Vector Concatenate1/3  "<OrientationYaw>"
  Bus Selector/5 -> Vector Concatenate1/2  "<OrientationPitch>"
  Bus Selector/4 -> Vector Concatenate1/1  "<OrientationRoll>"
  Vector Concatenate1/1 -> Gain/1
  Bus Selector/3 -> z [m]/1  "<PositionZ>"
  Bus Selector/2 -> y [m]/1  "<PositionY>"
  Bus Selector/1 -> x [m]/1  "<PositionX>"
  SELF/1 -> Bus Selector/1
  Gain/1 -> Demux2/1
  Demux2/1 -> rotx [deg]/1
  Demux2/2 -> roty [deg]/1
  Demux2/3 -> rotz [deg]/1
  compas converter/1(heading [deg]) -> heading [deg]/1
  Gain1/1 -> yaw rate [deg/s]/1

== system UberCase_cs/BMW_X5_1/ENABLED/STATE_BMW_X5_1 ==
  State : Inport  SampleTime=TimeStep
  Bus Creator : BusCreator  Inputs=15  OutDataTypeStr=Bus: PRESCAN_STATEACTUATORDATA  NonVirtualBus=on
  Demux : Demux  Outputs=15
  iniBODYAngles wrtVEH [rad] : Constant  Value=[Roll0 Pitch0 0]  SampleTime=TimeStep
  iniVEHAngles wrtGLOB [rad] : Constant  Value=[0 0 Yaw0]  SampleTime=TimeStep
  iniVEHposition wrtGLOB [m] : Constant  Value=[x0 y0 z0]  SampleTime=TimeStep
  state2FullState : PreScanSimulinkLibrary/state2FullState  SystemSampleTime=-1
  StateBus : Outport  OutDataTypeStr=Bus: PRESCAN_STATEACTUATORDATA
  wires:
  Bus Creator/1 -> StateBus/1
  State/1 -> state2FullState/1
  state2FullState/1 -> Demux/1
  iniVEHposition wrtGLOB [m]/1 -> state2FullState/2
  iniBODYAngles wrtVEH [rad]/1 -> state2FullState/3
  iniVEHAngles wrtGLOB [rad]/1 -> state2FullState/4
  Demux/1 -> Bus Creator/1  "PositionX"
  Demux/2 -> Bus Creator/2  "PositionY"
  Demux/3 -> Bus Creator/3  "PositionZ"
  Demux/4 -> Bus Creator/4  "VelocityX"
  Demux/5 -> Bus Creator/5  "VelocityY"
  Demux/6 -> Bus Creator/6  "VelocityZ"
  Demux/7 -> Bus Creator/7  "AccelerationX"
  Demux/8 -> Bus Creator/8  "AccelerationY"
  Demux/9 -> Bus Creator/9  "AccelerationZ"
  Demux/10 -> Bus Creator/10  "OrientationRoll"
  Demux/11 -> Bus Creator/11  "OrientationPitch"
  Demux/12 -> Bus Creator/12  "OrientationYaw"
  Demux/13 -> Bus Creator/13  "AngularVelocityRoll"
  Demux/14 -> Bus Creator/14  "AngularVelocityPitch"
  Demux/15 -> Bus Creator/15  "AngularVelocityYaw"

== system UberCase_cs/CollisionDetection/DISABLED/GND1 ==
  GND_DATA : Subsystem
  GND_HEADER : Subsystem
  buscreator : BusCreator  Inputs=2  OutDataTypeStr=Bus: PRESCAN_COLLISIONDETECTION_MESSAGE  NonVirtualBus=on
  concatenate : Concatenate  NumInputs=5
  bus : Outport  OutDataTypeStr=Bus: PRESCAN_COLLISIONDETECTION_MESSAGE
  wires:
  GND_HEADER/1(bus) -> buscreator/1  "HEADER"
  GND_DATA/1(bus) -> buscreator/2  "DATA"
  buscreator/1 -> concatenate/1, concatenate/2, concatenate/3, concatenate/4, concatenate/5
  concatenate/1 -> bus/1

== system UberCase_cs/Conventional_Car/DISABLED/GND1 ==
  GND_AccelerationX : Constant  Value=0
  GND_AccelerationY : Constant  Value=0
  GND_AccelerationZ : Constant  Value=0
  GND_AngularVelocityPitch : Constant  Value=0
  GND_AngularVelocityRoll : Constant  Value=0
  GND_AngularVelocityYaw : Constant  Value=0
  GND_OrientationPitch : Constant  Value=0
  GND_OrientationRoll : Constant  Value=0
  GND_OrientationYaw : Constant  Value=0
  GND_PositionX : Constant  Value=0
  GND_PositionY : Constant  Value=0
  GND_PositionZ : Constant  Value=0
  GND_VelocityX : Constant  Value=0
  GND_VelocityY : Constant  Value=0
  GND_VelocityZ : Constant  Value=0
  buscreator : BusCreator  Inputs=15  OutDataTypeStr=Bus: PRESCAN_STATEACTUATORDATA  NonVirtualBus=on
  bus : Outport  OutDataTypeStr=Bus: PRESCAN_STATEACTUATORDATA
  wires:
  GND_PositionX/1 -> buscreator/1  "PositionX"
  GND_PositionY/1 -> buscreator/2  "PositionY"
  GND_PositionZ/1 -> buscreator/3  "PositionZ"
  GND_VelocityX/1 -> buscreator/4  "VelocityX"
  GND_VelocityY/1 -> buscreator/5  "VelocityY"
  GND_VelocityZ/1 -> buscreator/6  "VelocityZ"
  GND_AccelerationX/1 -> buscreator/7  "AccelerationX"
  GND_AccelerationY/1 -> buscreator/8  "AccelerationY"
  GND_AccelerationZ/1 -> buscreator/9  "AccelerationZ"
  GND_OrientationRoll/1 -> buscreator/10  "OrientationRoll"
  GND_OrientationPitch/1 -> buscreator/11  "OrientationPitch"
  GND_OrientationYaw/1 -> buscreator/12  "OrientationYaw"
  GND_AngularVelocityRoll/1 -> buscreator/13  "AngularVelocityRoll"
  GND_AngularVelocityPitch/1 -> buscreator/14  "AngularVelocityPitch"
  GND_AngularVelocityYaw/1 -> buscreator/15  "AngularVelocityYaw"
  buscreator/1 -> bus/1

== system UberCase_cs/Conventional_Car/ENABLED/Camera_conventional_CM_Demux ==
  In1 : Inport
  Selector : Selector  NumberOfDimensions=2  InputPortWidth=3  IndexOptions=Index vector (dialog),Index vector (dialog)  Indices=-1,1:hres  OutputSizes=1,1
  Selector1 : Selector  NumberOfDimensions=2  InputPortWidth=3  IndexOptions=Index vector (dialog),Index vector (dialog)  Indices=-1,hres+1:hres*2  OutputSizes=1,1
  Selector2 : Selector  NumberOfDimensions=2  InputPortWidth=3  IndexOptions=Index vector (dialog),Index vector (dialog)  Indices=-1,hres*2+1:hres*3  OutputSizes=1,1
  R : Outport
  G : Outport  Port=2
  B : Outport  Port=3
  wires:
  In1/1 -> Selector1/1, Selector/1, Selector2/1
  Selector/1 -> R/1
  Selector1/1 -> G/1
  Selector2/1 -> B/1

== system UberCase_cs/Conventional_Car/ENABLED/SELF_Demux ==
  SELF : Inport  OutDataTypeStr=Bus: PRESCAN_SELFSENSORDATA
  Bus Selector : BusSelector  OutputSignals=PositionX,PositionY,PositionZ,OrientationRoll,OrientationPitch,OrientationYaw,Velocity,Yaw_rate,Lat,Long,Alt
  Demux2 : Demux  Outputs=3
  Gain : Gain  Gain=180/pi
  Gain1 : Gain  Gain=180/pi
  Vector Concatenate1 : Concatenate  NumInputs=3
  compas converter : Subsystem
  x [m] : Outport
  y [m] : Outport  Port=2
  z [m] : Outport  Port=3
  rotx [deg] : Outport  Port=4
  roty [deg] : Outport  Port=5
  rotz [deg] : Outport  Port=6
  GPS lat [deg] : Outport  Port=7
  GPS long [deg] : Outport  Port=8
  GPS alt [m] : Outport  Port=9
  velocity [m/s] : Outport  Port=10
  heading [deg] : Outport  Port=11
  yaw rate [deg/s] : Outport  Port=12
  wires:
  Bus Selector/11 -> GPS alt [m]/1  "<Alt>"
  Bus Selector/10 -> GPS long [deg]/1  "<Long>"
  Bus Selector/9 -> GPS lat [deg]/1  "<Lat>"
  Bus Selector/8 -> Gain1/1  "<Yaw_rate>"
  Bus Selector/7 -> velocity [m/s]/1  "<Velocity>"
  Bus Selector/6 -> compas converter/1(rotz [rad]), Vector Concatenate1/3  "<OrientationYaw>"
  Bus Selector/5 -> Vector Concatenate1/2  "<OrientationPitch>"
  Bus Selector/4 -> Vector Concatenate1/1  "<OrientationRoll>"
  Vector Concatenate1/1 -> Gain/1
  Bus Selector/3 -> z [m]/1  "<PositionZ>"
  Bus Selector/2 -> y [m]/1  "<PositionY>"
  Bus Selector/1 -> x [m]/1  "<PositionX>"
  SELF/1 -> Bus Selector/1
  Gain/1 -> Demux2/1
  Demux2/1 -> rotx [deg]/1
  Demux2/2 -> roty [deg]/1
  Demux2/3 -> rotz [deg]/1
  compas converter/1(heading [deg]) -> heading [deg]/1
  Gain1/1 -> yaw rate [deg/s]/1

== system UberCase_cs/Conventional_Car/ENABLED/STATE_Conventional_Car ==
  State : Inport  SampleTime=TimeStep
  Bus Creator : BusCreator  Inputs=15  OutDataTypeStr=Bus: PRESCAN_STATEACTUATORDATA  NonVirtualBus=on
  Demux : Demux  Outputs=15
  iniBODYAngles wrtVEH [rad] : Constant  Value=[Roll0 Pitch0 0]  SampleTime=TimeStep
  iniVEHAngles wrtGLOB [rad] : Constant  Value=[0 0 Yaw0]  SampleTime=TimeStep
  iniVEHposition wrtGLOB [m] : Constant  Value=[x0 y0 z0]  SampleTime=TimeStep
  state2FullState : PreScanSimulinkLibrary/state2FullState  SystemSampleTime=-1
  StateBus : Outport  OutDataTypeStr=Bus: PRESCAN_STATEACTUATORDATA
  wires:
  Bus Creator/1 -> StateBus/1
  State/1 -> state2FullState/1
  state2FullState/1 -> Demux/1
  iniVEHposition wrtGLOB [m]/1 -> state2FullState/2
  iniBODYAngles wrtVEH [rad]/1 -> state2FullState/3
  iniVEHAngles wrtGLOB [rad]/1 -> state2FullState/4
  Demux/1 -> Bus Creator/1  "PositionX"
  Demux/2 -> Bus Creator/2  "PositionY"
  Demux/3 -> Bus Creator/3  "PositionZ"
  Demux/4 -> Bus Creator/4  "VelocityX"
  Demux/5 -> Bus Creator/5  "VelocityY"
  Demux/6 -> Bus Creator/6  "VelocityZ"
  Demux/7 -> Bus Creator/7  "AccelerationX"
  Demux/8 -> Bus Creator/8  "AccelerationY"
  Demux/9 -> Bus Creator/9  "AccelerationZ"
  Demux/10 -> Bus Creator/10  "OrientationRoll"
  Demux/11 -> Bus Creator/11  "OrientationPitch"
  Demux/12 -> Bus Creator/12  "OrientationYaw"
  Demux/13 -> Bus Creator/13  "AngularVelocityRoll"
  Demux/14 -> Bus Creator/14  "AngularVelocityPitch"
  Demux/15 -> Bus Creator/15  "AngularVelocityYaw"
